simulink model "STOICAL_example_2"  (R2015b)
settings: Solver=ode4  StartTime=0.0  StopTime=1  FixedStep=50E-6  RelTol=1e-3
model workspace (MAT data in the model file):
  STOICAL.SignalSaveOptions.ReturnWorkspaceOutputs = 'on'
  STOICAL.SignalSaveOptions.ReturnWorkspaceOutputsName = 'simout_obj'
  STOICAL.SignalSaveOptions.SignalLogging = 'on'
  STOICAL.SignalSaveOptions.SignalLoggingSaveFormat = 'Dataset'
  STOICAL.SignalSaveOptions.SignalLoggingName = 'STOVICAL_LoggedSignals'
  STOICAL.ParameterDefinition.BlkNameFull{1} = 'Step amplitude
    | #PARAM#Amplitude'
  STOICAL.ParameterDefinition.BlkNameFull{2} = 'Dynamic System
    | #PARAM#w0#damp'
  STOICAL.ParameterDefinition.BlkNameFull{3} = 'Static System
    | modelled
    | by gain block
    | #PARAM#SystemGain'
  STOICAL.ParameterDefinition.BlkNameFull{4} = 'Dynamic System
    | #PARAM#w0#damp'
  STOICAL.ParameterDefinition.BlkNameShort{1} = 'Step amplitude
    | '
  STOICAL.ParameterDefinition.BlkNameShort{2} = 'Dynamic System
    | '
  STOICAL.ParameterDefinition.BlkNameShort{3} = 'Static System
    | modelled
    | by gain block
    | '
  STOICAL.ParameterDefinition.BlkNameShort{4} = 'Dynamic System
    | '
  STOICAL.ParameterDefinition.BlkHandle = [8.0009765625; 15.0009765625; 21.0024414062; 15.0009765625]
  STOICAL.ParameterDefinition.ParamName = {'Amplitude'; 'w0'; 'SystemGain'; 'damp'}
  STOICAL.ParameterDefinition.BlkPath{1} = 'STOICAL_example_2_Step03_Activation/#UNIT#Stimulus/Step amplitude
    | #PARAM#Amplitude'
  STOICAL.ParameterDefinition.BlkPath{2} = 'STOICAL_example_2_Step03_Activation/#UNIT#System/Dynamic System
    | #PARAM#w0#damp'
  STOICAL.ParameterDefinition.BlkPath{3} = 'STOICAL_example_2_Step03_Activation/#UNIT#System/Static System
    | modelled
    | by gain block
    | #PARAM#SystemGain'
  STOICAL.ParameterDefinition.BlkPath{4} = 'STOICAL_example_2_Step03_Activation/#UNIT#System/Dynamic System
    | #PARAM#w0#damp'
  STOICAL.ParameterDefinition.BlkType = {'Constant'; 'SubSystem'; 'Gain'; 'SubSystem'}
  STOICAL.ParameterDefinition.BlkMaskType = {''; ''; ''; ''}
  STOICAL.ParameterDefinition.ParentalBlockPath = {'STOICAL_example_2_Step03_Activation/#UNIT#Stimulus'; 'STOICAL_example_2_Step03_Activation/#UNIT#System'; 'STOICAL_example_2_Step03_Activation/#UNIT#System'; 'STOICAL_example_2_Step03_Activation/#UNIT#System'}
  STOICAL.ParameterDefinition.ParentalBlockHandle = [5.02294921875; 13.0029296875; 13.0029296875; 13.0029296875]
  STOICAL.ParameterDefinition.Belongs2SubsystemHdl = [5.02294921875; 15.0009765625; 13.0029296875; 15.0009765625]
  STOICAL.ParameterDefinition.NrParams = 4
  STOICAL.ParameterDefinition.BlkField2Set = {'Value'; 'w0'; 'Gain'; 'damp'}
  STOICAL.ParameterDefinition.BlkFieldSyntax = {'#'; '#'; '#'; '#'}
  STOICAL.ParameterDefinition.ParamVariable = {'param_9ba35cf139ae8d049712606822772694'; 'param_518f5dd230dc6df197dc8805b8657145'; 'param_b7a2875e19f2aaba8a6b37e383b6fdf1'; 'param_13ac9ebe924e8dfd32ee0d3deb3cd2af'}
  STOICAL.ParameterDefinition.LabelPath = {'#Stimulus#Amplitude'; '#System#w0'; '#System#SystemGain'; '#System#damp'}
  STOICAL.ParameterDefinition.ParamDefaultValue = {'2'; '50'; '5'; '1/sqrt(2)'}
  STOICAL.SignalDefinition.ParentalBlockPath = {'STOICAL_example_2_Step03_Activation'; 'STOICAL_example_2_Step03_Activation'}
  STOICAL.SignalDefinition.ParentalBlockHandle = [3.0009765625; 3.0009765625]
  STOICAL.SignalDefinition.NameInDiagram = {'#SIG#stimulus'; '#SIG#response'}
  STOICAL.SignalDefinition.SourceBlockPath = {'STOICAL_example_2_Step03_Activation/#UNIT#Stimulus'; 'STOICAL_example_2_Step03_Activation/#UNIT#System'}
  STOICAL.SignalDefinition.SourceBlockPort = [1; 1]
  STOICAL.SignalDefinition.SourceBlockHandle = [5.02294921875; 13.0029296875]
  STOICAL.SignalDefinition.Handle = [1948.00146484; 1949.01672363]
  STOICAL.SignalDefinition.NrSig = 2
  STOICAL.SignalDefinition.NameOfLogVar = {'logsig_643e3731b0c65fb38afb5e4f06d06a3f'; 'logsig_ee10c39bc06b89f4e4e488efcbc6167c'}
  STOICAL.SignalDefinition.NameOfLogVarMode = {'Custom'; 'Custom'}
  STOICAL.SignalDefinition.DoLog = [1; 1]
  STOICAL.SignalDefinition.LabelPath = {'#stimulus'; '#response'}
  STOICAL.VariantDefinition.NodeHandle = [3.0009765625; 5.02294921875; 13.0029296875; 15.0009765625]
  STOICAL.VariantDefinition.NodeName{1} = 'STOICAL_example_2_Step03_Activation'
  STOICAL.VariantDefinition.NodeName{2} = '#UNIT#Stimulus'
  STOICAL.VariantDefinition.NodeName{3} = '#UNIT#System'
  STOICAL.VariantDefinition.NodeName{4} = 'Dynamic System
    | #PARAM#w0#damp'
  STOICAL.VariantDefinition.IsVariantSubsystem = [0; 0; 0; 0]
  STOICAL.VariantDefinition.NodeLevel = [1; 2; 2; 3]
  STOICAL.VariantDefinition.NodePath{1} = 'STOICAL_example_2_Step03_Activation'
  STOICAL.VariantDefinition.NodePath{2} = 'STOICAL_example_2_Step03_Activation/#UNIT#Stimulus'
  STOICAL.VariantDefinition.NodePath{3} = 'STOICAL_example_2_Step03_Activation/#UNIT#System'
  STOICAL.VariantDefinition.NodePath{4} = 'STOICAL_example_2_Step03_Activation/#UNIT#System/Dynamic System
    | #PARAM#w0#damp'
  STOICAL.VariantDefinition.IsVariant = [0; 0; 0; 0]
  STOICAL.VariantDefinition.VSNodeIdxofVariant = [0; 0; 0; 0]
  STOICAL.VariantDefinition.VSVariantsCount = [0; 0; 0; 0]
  STOICAL.VariantDefinition.VSVariantsBlkHdls = {[]; []; []; []}
  STOICAL.VariantDefinition.VSVariantsNodeIdx = {[]; []; []; []}
  STOICAL.VariantDefinition.VSControlVariable = {[]; []; []; []}
  STOICAL.VariantDefinition.VSVariantHasNr = [0; 0; 0; 0]
  STOICAL.VariantDefinition.LabelPath = {[]; []; []; []}
  param_13ac9ebe924e8dfd32ee0d3deb3cd2af = '1/sqrt(2)'
  param_518f5dd230dc6df197dc8805b8657145 = '50'
  param_9ba35cf139ae8d049712606822772694 = '2'
  param_afc1e04cc1c158b687408e5b6ea19d06 = '5'
  param_b7a2875e19f2aaba8a6b37e383b6fdf1 = '5'
  param_ec6e274da2c23e664dfdc874ac252818 = '2'
settings Model: Creator=Wippenbeck  LastModifiedBy=bertram
settings DataIOCC: SaveFormat=Array  ReturnWorkspaceOutputs=on  SignalLoggingName=STOVICAL_LoggedSignals  ReturnWorkspaceOutputsName=simout_obj
settings DebuggingCC: SolverPrmCheckMsg=warning
settings HardwareCC: ProdBitPerPointer=32  ProdLargestAtomicFloat=None  ProdIntDivRoundTo=Undefined  ProdEndianess=Unspecified  ProdWordSize=32  ProdHWDeviceType=32-bit Generic
settings GRTTargetCC: GeneratePreprocessorConditionals=Disable all
settings ConfigComp: CovModelRefEnable=Off  CovSFcnEnable=off

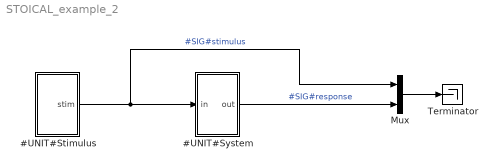
== system STOICAL_example_2 ==
  #UNIT#Stimulus : Subsystem
  #UNIT#System : Subsystem
  Mux : Mux  Inputs=2
  Terminator : Terminator
  wires:
  Mux/1 -> Terminator/1
  #UNIT#Stimulus/1(stim) -> #UNIT#System/1(in), Mux/1  "#SIG#stimulus"
  #UNIT#System/1(out) -> Mux/2  "#SIG#response"

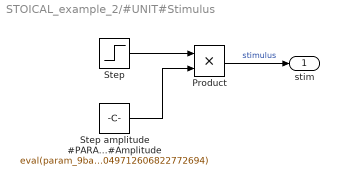
== system STOICAL_example_2/#UNIT#Stimulus ==
  Product : Product
  Step : Step  Time=0.1  SampleTime=0
  Step amplitude #PARAM#Amplitude : Constant  Value=eval(param_9ba35cf139ae8d049712606822772694)
  stim : Outport
  wires:
  Step amplitude #PARAM#Amplitude/1 -> Product/2
  Product/1 -> stim/1  "stimulus"
  Step/1 -> Product/1

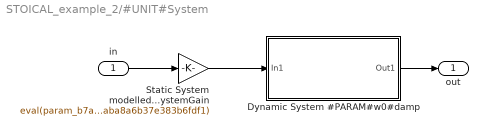
== system STOICAL_example_2/#UNIT#System ==
  in : Inport
  Dynamic System #PARAM#w0#damp : Subsystem  mask{w0=eval(param_518f5dd230dc6df197dc8805b8657145), damp=eval(param_13ac9ebe924e8dfd32ee0d3deb3cd2af)}
      mask prompts: w0 "Natural frequency w0 [rad/s]"; damp "Damping zeta [1]"
      mask help:
      | Dynamical system of the form
      |
      | G(s) = w0^2 / (s^2 + 2*zeta*w0*s + wo^2)
  Static System modelled by gain block #PARAM#SystemGain : Gain  Gain=eval(param_b7a2875e19f2aaba8a6b37e383b6fdf1)
  out : Outport
  wires:
  in/1 -> Static System modelled by gain block #PARAM#SystemGain/1
  Static System modelled by gain block #PARAM#SystemGain/1 -> Dynamic System #PARAM#w0#damp/1(In1)
  Dynamic System #PARAM#w0#damp/1(Out1) -> out/1

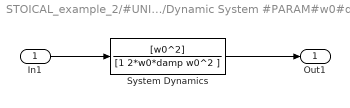
== system STOICAL_example_2/#UNIT#System/Dynamic System #PARAM#w0#damp ==
  In1 : Inport
  System Dynamics : TransferFcn  Numerator=[w0^2]  Denominator=[1 2*w0*damp w0^2 ]
  Out1 : Outport
  wires:
  System Dynamics/1 -> Out1/1
  In1/1 -> System Dynamics/1
